simulink model "pitch_control_simulink"  (R2023a)
settings: Solver=VariableStepAuto  StartTime=0.0  StopTime=300  RelTol=1e-3
values from neighbouring files (symbols this model uses):
  C_D = 0.1    [variables.m]
  C_L = 0.034    [variables.m]
  g = 9.81    [variables.m]
  I_sp0 = 300    [variables.m]
  I_y = 3100    [variables.m]
  k_1_theta = 12    [variables.m]
  k_1_x = 2.5    [variables.m]
  k_2_theta = 10    [variables.m]
  k_2_x = 4.5    [variables.m]
  k_i = 0.13    [variables.m]
  k_z = 0.61    [variables.m]
  k_z_dot = 1.11    [variables.m]
  l = 4.18    [variables.m]
  m_0 = 1250.0    (= 1250)    [variables.m]
  x_cm = 4.18    [variables.m]
  x_cp = 7.11    [variables.m]
settings Model: Creator=nicla  LastModifiedBy=nicla

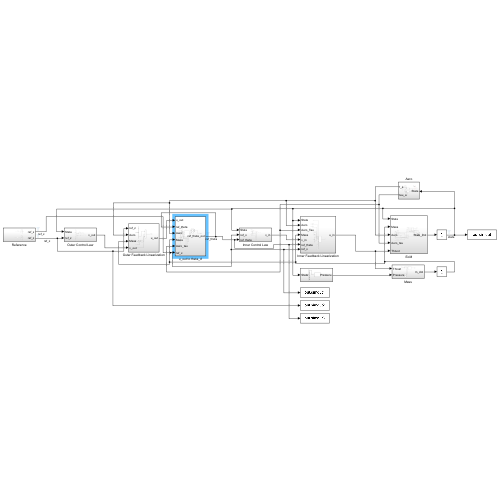
[thumbnail: Simulink's stored preview of the top-level diagram]
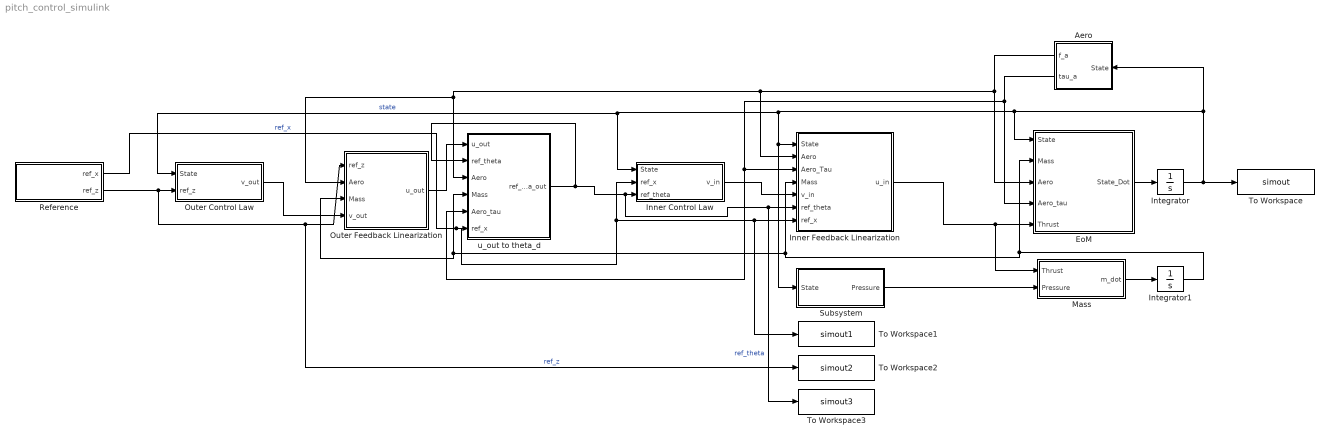
== system pitch_control_simulink ==
  Aero : Subsystem
  EoM : Subsystem
  Inner Control Law : Subsystem
  Inner Feedback Linearization : Subsystem
  Integrator : Integrator
  Integrator1 : Integrator  InitialCondition=m_0
  Mass : Subsystem
  Outer Control Law : Subsystem
  Outer Feedback Linearization : Subsystem
  Reference : Subsystem
  Subsystem : Subsystem
  To Workspace : ToWorkspace  VariableName=simout  SaveFormat=Timeseries  SampleTime=-1
  To Workspace1 : ToWorkspace  VariableName=simout1  SaveFormat=Timeseries  SampleTime=-1
  To Workspace2 : ToWorkspace  VariableName=simout2  SaveFormat=Timeseries  SampleTime=-1
  To Workspace3 : ToWorkspace  VariableName=simout3  SaveFormat=Timeseries  SampleTime=-1
  u_out to theta_d : Subsystem
  wires:
  EoM/1(State_Dot) -> Integrator/1
  Inner Feedback Linearization/1(u_in) -> Mass/1(Thrust), EoM/5(Thrust)
  Inner Control Law/1(v_in) -> Inner Feedback Linearization/5(v_in)
  Integrator/1 -> To Workspace/1, Outer Control Law/1(State), Inner Control Law/1(State), Subsystem/1(State), Inner Feedback Linearization/1(State), EoM/1(State), Aero/1(State)  "state"
  Aero/1(f_a) -> Outer Feedback Linearization/2(Aero), u_out to theta_d/3(Aero), Inner Feedback Linearization/2(Aero), EoM/3(Aero)
  Aero/2(tau_a) -> u_out to theta_d/5(Aero_tau), Inner Feedback Linearization/3(Aero_Tau), EoM/4(Aero_tau)
  Mass/1(m_dot) -> Integrator1/1
  Integrator1/1 -> EoM/2(Mass), Outer Feedback Linearization/3(Mass), u_out to theta_d/4(Mass), Inner Feedback Linearization/4(Mass)
  Subsystem/1(Pressure) -> Mass/2(Pressure)
  Outer Feedback Linearization/1(u_out) -> u_out to theta_d/1(u_out)
  Outer Control Law/1(v_out) -> Outer Feedback Linearization/4(v_out)
  Reference/2(ref_z) -> To Workspace2/1, Outer Feedback Linearization/1(ref_z), Outer Control Law/2(ref_z)  "ref_z"
  Reference/1(ref_x) -> Inner Control Law/2(ref_x), To Workspace1/1, Inner Feedback Linearization/7(ref_x), u_out to theta_d/6(ref_x)  "ref_x"
  u_out to theta_d/1(ref_theta_out) -> u_out to theta_d/2(ref_theta), To Workspace3/1, Inner Feedback Linearization/6(ref_theta), Inner Control Law/3(ref_theta)  "ref_theta"

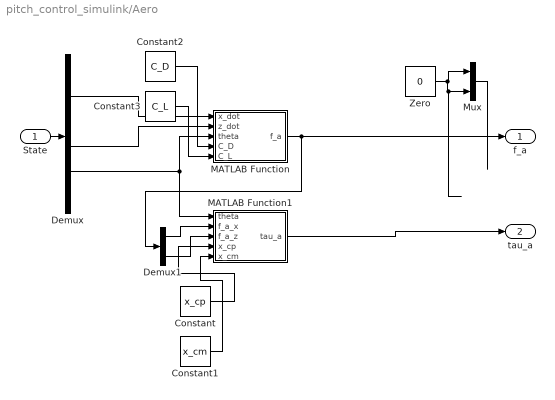
== system pitch_control_simulink/Aero ==
  State : Inport
  Constant : Constant  Value=x_cp
  Constant1 : Constant  Value=x_cm
  Constant2 : Constant  Value=C_D
  Constant3 : Constant  Value=C_L
  Demux : Demux  Outputs=6
  Demux1 : Demux  Outputs=2
  MATLAB Function : MATLAB Function  TreatAsAtomicUnit=on
  MATLAB Function1 : MATLAB Function  TreatAsAtomicUnit=on
  Mux : Mux  Inputs=2
  Zero : Constant  Value=0  OutDataTypeStr=Inherit: Inherit via back propagation
  f_a : Outport
  tau_a : Outport  Port=2
  wires:
  State/1 -> Demux/1
  Demux/2 -> MATLAB Function/1(x_dot)
  Demux/4 -> MATLAB Function/2(z_dot)
  Demux/5 -> MATLAB Function/3(theta), MATLAB Function1/1(theta)
  MATLAB Function/1(f_a) -> f_a/1, Demux1/1
  Demux1/1 -> MATLAB Function1/2(f_a_x)
  Demux1/2 -> MATLAB Function1/3(f_a_z)
  MATLAB Function1/1(tau_a) -> tau_a/1
  Constant/1 -> MATLAB Function1/4(x_cp)
  Constant1/1 -> MATLAB Function1/5(x_cm)
  Constant2/1 -> MATLAB Function/4(C_D)
  Constant3/1 -> MATLAB Function/5(C_L)
  Zero/1 -> Mux/2, Mux/1
  Mux/1 -> ?

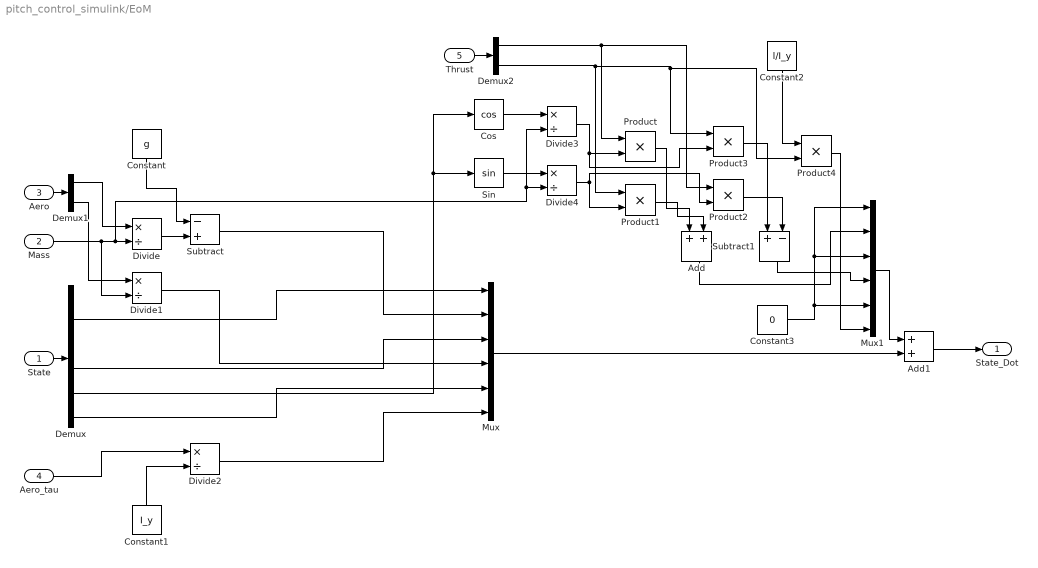
== system pitch_control_simulink/EoM ==
  State : Inport
  Mass : Inport  Port=2
  Aero : Inport  Port=3
  Aero_tau : Inport  Port=4
  Thrust : Inport  Port=5
  Add : Sum
  Add1 : Sum
  Constant : Constant  Value=g
  Constant1 : Constant  Value=I_y
  Constant2 : Constant  Value=l/I_y
  Constant3 : Constant  Value=0
  Cos : Trigonometry  Operator=cos
  Demux : Demux  Outputs=6
  Demux1 : Demux  Outputs=2
  Demux2 : Demux  Outputs=2
  Divide{,1..4} (5 alike) : Product  Inputs=*/
  Mux : Mux  Inputs=6
  Mux1 : Mux  Inputs=6
  Product{,1..4} (5 alike) : Product
  Sin : Trigonometry
  Subtract : Sum  Inputs=-+
  Subtract1 : Sum  Inputs=+-
  State_Dot : Outport
  wires:
  State/1 -> Demux/1
  Demux/2 -> Mux/1
  Aero/1 -> Demux1/1
  Demux1/1 -> Divide/1
  Mass/1 -> Divide1/2, Divide3/2, Divide4/2, Divide/2
  Divide/1 -> Subtract/2
  Constant/1 -> Subtract/1
  Subtract/1 -> Mux/2
  Demux/4 -> Mux/3
  Demux/6 -> Mux/5
  Demux1/2 -> Divide1/1
  Divide1/1 -> Mux/4
  Constant1/1 -> Divide2/2
  Aero_tau/1 -> Divide2/1
  Divide2/1 -> Mux/6
  Thrust/1 -> Demux2/1
  Demux/5 -> Cos/1, Sin/1
  Cos/1 -> Divide3/1
  Sin/1 -> Divide4/1
  Demux2/1 -> Product2/1, Product/1
  Divide3/1 -> Product3/2, Product/2
  Divide4/1 -> Product2/2, Product1/2
  Demux2/2 -> Product4/2, Product3/1, Product1/1
  Product/1 -> Add/1
  Product1/1 -> Add/2
  Product2/1 -> Subtract1/2
  Product3/1 -> Subtract1/1
  Constant2/1 -> Product4/1
  Add/1 -> Mux1/2
  Subtract1/1 -> Mux1/4
  Product4/1 -> Mux1/6
  Constant3/1 -> Mux1/1, Mux1/3, Mux1/5
  Mux1/1 -> Add1/1
  Mux/1 -> Add1/2
  Add1/1 -> State_Dot/1

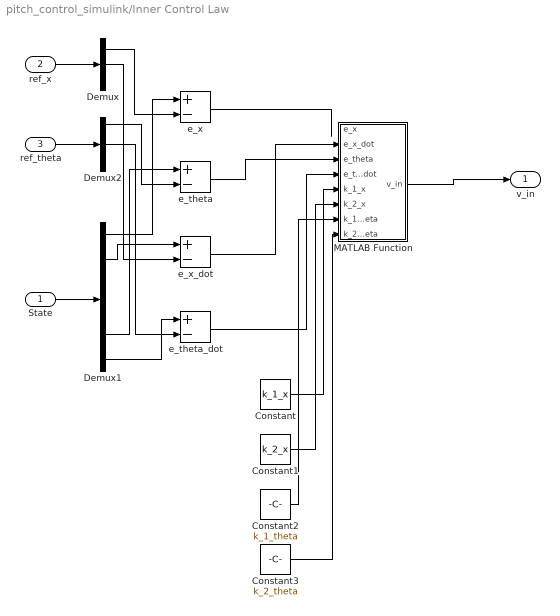
== system pitch_control_simulink/Inner Control Law ==
  State : Inport
  ref_x : Inport  Port=2
  ref_theta : Inport  Port=3
  Constant : Constant  Value=k_1_x
  Constant1 : Constant  Value=k_2_x
  Constant2 : Constant  Value=k_1_theta
  Constant3 : Constant  Value=k_2_theta
  Demux : Demux  Outputs=3
  Demux1 : Demux  Outputs=6
  Demux2 : Demux  Outputs=3
  MATLAB Function : MATLAB Function  TreatAsAtomicUnit=on
  e_theta : Sum  Inputs=+-
  e_theta_dot : Sum  Inputs=+-
  e_x : Sum  Inputs=+-
  e_x_dot : Sum  Inputs=+-
  v_in : Outport
  wires:
  ref_x/1 -> Demux/1
  State/1 -> Demux1/1
  Demux1/1 -> e_x/1
  Demux/1 -> e_x/2
  Demux1/5 -> e_theta/1
  Demux2/1 -> e_theta/2
  Demux1/2 -> e_x_dot/1
  Demux/2 -> e_x_dot/2
  Demux2/2 -> e_theta_dot/2
  Demux1/6 -> e_theta_dot/1
  MATLAB Function/1(v_in) -> v_in/1
  e_x_dot/1 -> MATLAB Function/2(e_x_dot)
  e_x/1 -> ?
  e_theta/1 -> MATLAB Function/3(e_theta)
  e_theta_dot/1 -> MATLAB Function/4(e_theta_dot)
  ref_theta/1 -> Demux2/1
  Constant/1 -> MATLAB Function/5(k_1_x)
  Constant1/1 -> MATLAB Function/6(k_2_x)
  Constant2/1 -> MATLAB Function/7(k_1_theta)
  Constant3/1 -> MATLAB Function/8(k_2_theta)

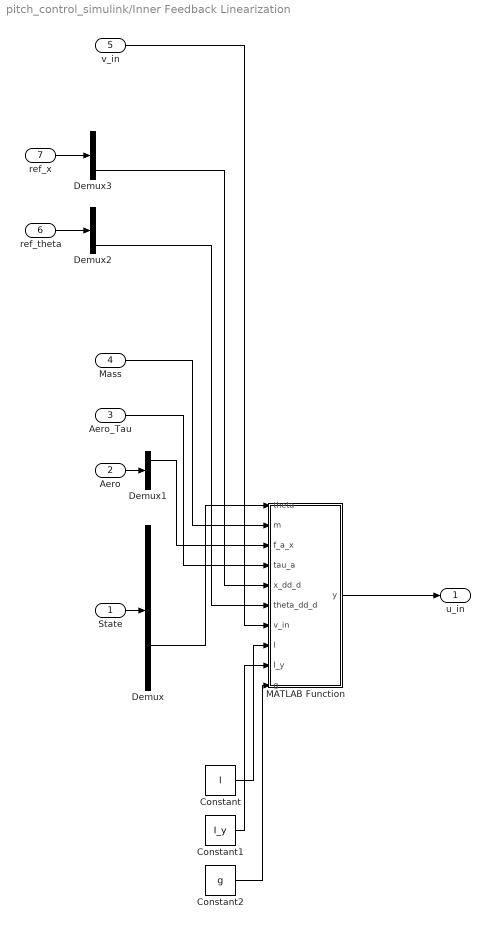
== system pitch_control_simulink/Inner Feedback Linearization ==
  State : Inport
  Aero : Inport  Port=2
  Aero_Tau : Inport  Port=3
  Mass : Inport  Port=4
  v_in : Inport  Port=5
  ref_theta : Inport  Port=6
  ref_x : Inport  Port=7
  Constant : Constant  Value=l
  Constant1 : Constant  Value=I_y
  Constant2 : Constant  Value=g
  Demux : Demux  Outputs=6
  Demux1 : Demux  Outputs=2
  Demux2 : Demux  Outputs=3
  Demux3 : Demux  Outputs=3
  MATLAB Function : MATLAB Function  TreatAsAtomicUnit=on
  u_in : Outport
  wires:
  State/1 -> Demux/1
  Demux/5 -> MATLAB Function/1(theta)
  Aero/1 -> Demux1/1
  Mass/1 -> MATLAB Function/2(m)
  Aero_Tau/1 -> MATLAB Function/4(tau_a)
  Demux1/1 -> MATLAB Function/3(f_a_x)
  Demux3/3 -> MATLAB Function/5(x_dd_d)
  Demux2/3 -> MATLAB Function/6(theta_dd_d)
  v_in/1 -> MATLAB Function/7(v_in)
  MATLAB Function/1(y) -> u_in/1
  ref_theta/1 -> Demux2/1
  ref_x/1 -> Demux3/1
  Constant/1 -> MATLAB Function/8(l)
  Constant1/1 -> MATLAB Function/9(I_y)
  Constant2/1 -> MATLAB Function/10(g)

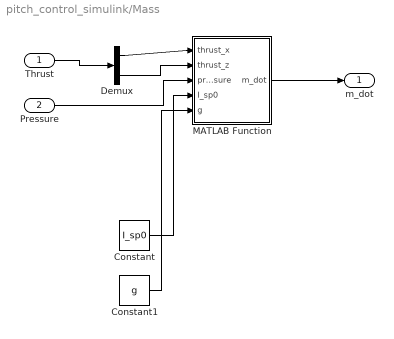
== system pitch_control_simulink/Mass ==
  Thrust : Inport
  Pressure : Inport  Port=2
  Constant : Constant  Value=I_sp0
  Constant1 : Constant  Value=g
  Demux : Demux  Outputs=2
  MATLAB Function : MATLAB Function  TreatAsAtomicUnit=on
  m_dot : Outport
  wires:
  Demux/2 -> MATLAB Function/2(thrust_z)
  Demux/1 -> MATLAB Function/1(thrust_x)
  Thrust/1 -> Demux/1
  Pressure/1 -> MATLAB Function/3(pressure)
  MATLAB Function/1(m_dot) -> m_dot/1
  Constant/1 -> MATLAB Function/4(I_sp0)
  Constant1/1 -> MATLAB Function/5(g)

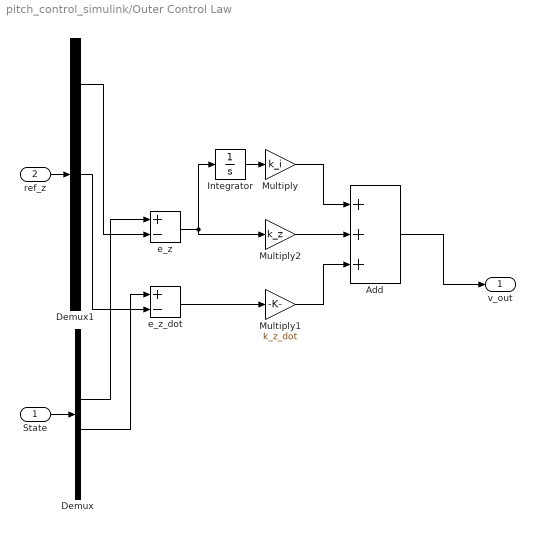
== system pitch_control_simulink/Outer Control Law ==
  State : Inport
  ref_z : Inport  Port=2
  Add : Sum  Inputs=+++
  Demux : Demux  Outputs=6
  Demux1 : Demux  Outputs=3
  Integrator : Integrator
  Multiply : Gain  Gain=k_i
  Multiply1 : Gain  Gain=k_z_dot
  Multiply2 : Gain  Gain=k_z
  e_z : Sum  Inputs=+-
  e_z_dot : Sum  Inputs=+-
  v_out : Outport
  wires:
  State/1 -> Demux/1
  ref_z/1 -> Demux1/1
  Demux/3 -> e_z/1
  Demux1/1 -> e_z/2
  Demux/4 -> e_z_dot/1
  Demux1/2 -> e_z_dot/2
  e_z/1 -> Integrator/1, Multiply2/1
  e_z_dot/1 -> Multiply1/1
  Integrator/1 -> Multiply/1
  Multiply2/1 -> Add/2
  Multiply/1 -> Add/1
  Multiply1/1 -> Add/3
  Add/1 -> v_out/1

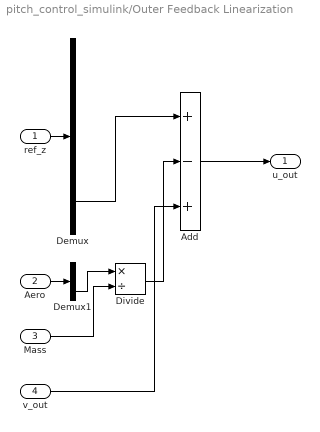
== system pitch_control_simulink/Outer Feedback Linearization ==
  ref_z : Inport
  Aero : Inport  Port=2
  Mass : Inport  Port=3
  v_out : Inport  Port=4
  Add : Sum  Inputs=+-+
  Demux : Demux  Outputs=3
  Demux1 : Demux  Outputs=2
  Divide : Product  Inputs=*/
  u_out : Outport
  wires:
  ref_z/1 -> Demux/1
  Demux/3 -> Add/1
  Aero/1 -> Demux1/1
  Demux1/2 -> Divide/1
  Mass/1 -> Divide/2
  Divide/1 -> Add/2
  v_out/1 -> Add/3
  Add/1 -> u_out/1

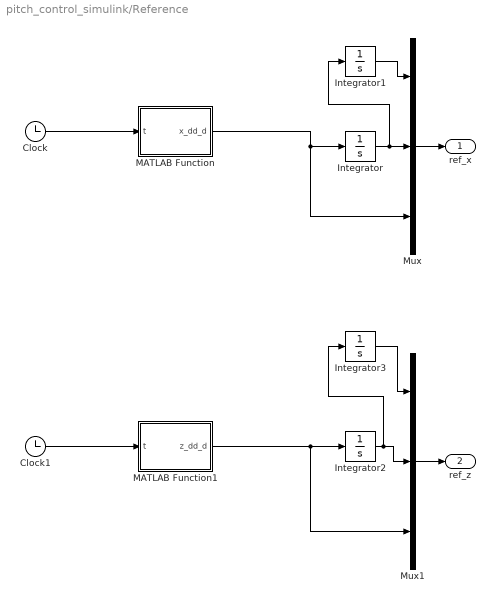
== system pitch_control_simulink/Reference ==
  Clock : Clock
  Clock1 : Clock
  Integrator{,1..3} (4 alike) : Integrator
  MATLAB Function : MATLAB Function  TreatAsAtomicUnit=on
  MATLAB Function1 : MATLAB Function  TreatAsAtomicUnit=on
  Mux : Mux  Inputs=3
  Mux1 : Mux  Inputs=3
  ref_x : Outport
  ref_z : Outport  Port=2
  wires:
  Clock/1 -> MATLAB Function/1(t)
  Mux/1 -> ref_x/1
  MATLAB Function/1(x_dd_d) -> Integrator/1, Mux/3
  Integrator/1 -> Integrator1/1, Mux/2
  Integrator1/1 -> Mux/1
  Mux1/1 -> ref_z/1
  MATLAB Function1/1(z_dd_d) -> Integrator2/1, Mux1/3
  Clock1/1 -> MATLAB Function1/1(t)
  Integrator3/1 -> Mux1/1
  Integrator2/1 -> Integrator3/1, Mux1/2

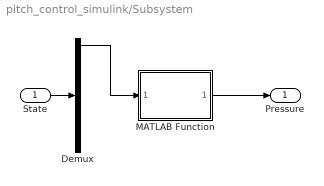
== system pitch_control_simulink/Subsystem ==
  State : Inport
  Demux : Demux  Outputs=6
  MATLAB Function : MATLAB Function  TreatAsAtomicUnit=on
  Pressure : Outport
  wires:
  State/1 -> Demux/1
  MATLAB Function/1(pressure) -> Pressure/1
  Demux/1 -> MATLAB Function/1(altitude)

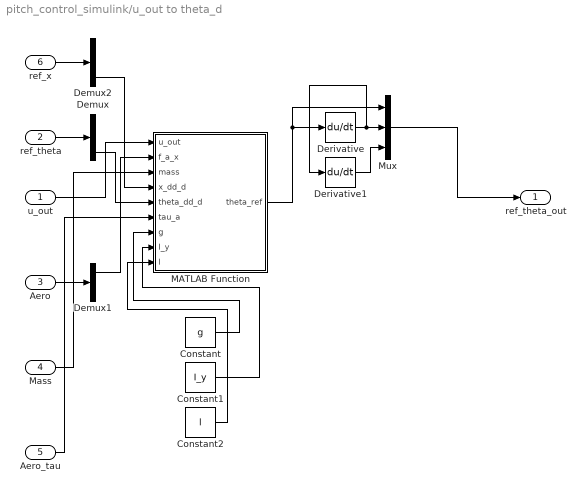
== system pitch_control_simulink/u_out to theta_d ==
  u_out : Inport
  ref_theta : Inport  Port=2
  Aero : Inport  Port=3
  Mass : Inport  Port=4
  Aero_tau : Inport  Port=5
  ref_x : Inport  Port=6
  Constant : Constant  Value=g
  Constant1 : Constant  Value=I_y
  Constant2 : Constant  Value=l
  Demux : Demux  Outputs=3
  Demux1 : Demux  Outputs=2
  Demux2 : Demux  Outputs=3
  Derivative : Derivative
  Derivative1 : Derivative
  MATLAB Function : MATLAB Function  TreatAsAtomicUnit=on
  Mux : Mux  Inputs=3
  ref_theta_out : Outport
  wires:
  ref_theta/1 -> Demux/1
  Aero/1 -> Demux1/1
  u_out/1 -> MATLAB Function/1(u_out)
  Demux1/1 -> MATLAB Function/2(f_a_x)
  Mass/1 -> MATLAB Function/3(mass)
  Demux/3 -> MATLAB Function/5(theta_dd_d)
  Aero_tau/1 -> MATLAB Function/6(tau_a)
  MATLAB Function/1(theta_ref) -> Mux/1, Derivative/1
  Derivative/1 -> Derivative1/1, Mux/2
  Derivative1/1 -> Mux/3
  Mux/1 -> ref_theta_out/1
  ref_x/1 -> Demux2/1
  Demux2/3 -> MATLAB Function/4(x_dd_d)
  Constant/1 -> MATLAB Function/7(g)
  Constant1/1 -> MATLAB Function/8(I_y)
  Constant2/1 -> MATLAB Function/9(l)

== matlab function pitch_control_simulink/Reference/MATLAB Function ==
  data: t input; x_dd_d output
function x_dd_d = x_dd_ref(t)
    if t < 0
        x_dd_d = 0.0;
    elseif t <= 30.0
        x_dd_d = 10.0;
    elseif t <= 60.0
        x_dd_d = 2.5 * cos(2 * pi * t / 30.0);
    else
        x_dd_d = 10.0;
    end
end

== matlab function pitch_control_simulink/Reference/MATLAB Function1 ==
  data: t input; z_dd_d output
function z_dd_d = z_dd_ref(t)
    if t < 20.0
        z_dd_d = 0.0;
    elseif t <= 60.0
        z_dd_d = 2.5 * cos(2*pi*t/40.0) + 2.5;
    else
        z_dd_d = 0.0
    end
end

== matlab function pitch_control_simulink/Inner Control Law/MATLAB Function ==
  data: e_x input; v_in output; e_x_dot input; e_theta input; e_theta_dot input; k_1_x input; k_2_x input; k_1_theta input; k_2_theta input
function v_in = fcn(e_x, e_x_dot, e_theta, e_theta_dot, k_1_x, k_2_x, k_1_theta, k_2_theta)
    v_in = [-(1 + k_1_x*k_2_x)*e_x - (k_1_x + k_2_x)*e_x_dot;
        -(1 + k_1_theta*k_2_theta)*e_theta - (k_1_theta + k_2_theta)*e_theta_dot];

== matlab function pitch_control_simulink/Inner Feedback Linearization/MATLAB Function ==
  data: theta input; y output; m input; f_a_x input; tau_a input; x_dd_d input; theta_dd_d input; v_in input; l input; I_y input; g input
function y = u_in(theta, m, f_a_x, tau_a, x_dd_d, theta_dd_d, v_in, l, I_y, g)
    Lambda = [cos(theta)/m, sin(theta)/m; 0, l/I_y];
    b = [-g + f_a_x/m - x_dd_d; tau_a/I_y - theta_dd_d];

    u_in = -inv(Lambda)*b + inv(Lambda)*v_in;
y = u_in

== matlab function pitch_control_simulink/Aero/MATLAB Function ==
  data: x_dot input; f_a output; z_dot input; theta input; C_D input; C_L input
function f_a = aero(x_dot, z_dot, theta, C_D, C_L)
    velocity = sqrt(x_dot^2 + z_dot^2);
    q_dyn = 0.5*1.225*velocity^2;

    gamma = atan2(z_dot, x_dot);
    alpha = theta - gamma;

    C_A = C_D*cos(alpha) - C_L*sin(alpha);
    C_N = C_L*cos(alpha) + C_D*sin(alpha);

    S = pi*0.5^2;

    F_A = -q_dyn*C_A*S;
    F_N = -q_dyn*C_N*S;

    f_a = [cos(theta), sin(theta); -sin(theta), cos(theta)]*[F_A; F_N];

== matlab function pitch_control_simulink/Aero/MATLAB Function1 ==
  data: theta input; tau_a output; f_a_x input; f_a_z input; x_cp input; x_cm input
function tau_a = aero_tau(theta, f_a_x, f_a_z, x_cp, x_cm)
    R = [cos(theta), sin(theta); -sin(theta), cos(theta)];
    f_body = R'*[f_a_x; f_a_z];
    f_az_body = f_body(2);
    
    tau_a = f_az_body*(x_cp - x_cm);

== matlab function pitch_control_simulink/Mass/MATLAB Function ==
  data: thrust_x input; m_dot output; thrust_z input; pressure input; I_sp0 input; g input
function m_dot = mass_fcn(thrust_x, thrust_z, pressure, I_sp0, g)
    T = sqrt(thrust_x^2 + thrust_z^2);

    m_dot = -T/(I_sp0*g) - (pressure * pi * 0.5^2)/(I_sp0*g);

== matlab function pitch_control_simulink/Subsystem/MATLAB Function ==
  data: altitude input; pressure output
function pressure = pressure_altitude(altitude)
    pressure = 101325*exp(-altitude/8500);

== matlab function pitch_control_simulink/u_out to theta_d/MATLAB Function ==
  data: u_out input; theta_ref output; f_a_x input; mass input; x_dd_d input; theta_dd_d input; tau_a input; g input; I_y input; l input
function theta_ref = u_out_to_theta_ref(u_out, f_a_x, mass, x_dd_d, theta_dd_d, tau_a, g, I_y, l)
    a = -g + f_a_x/mass - x_dd_d;
    b = (I_y*theta_dd_d - tau_a)/(mass*l);

    ratio = b / sqrt(a^2 + u_out^2);
    ratio = max(min(ratio, 1), -1); % Clamp the value between -1 and 1
    theta_ref = acos(ratio) + atan2(a, -u_out);
